simulink model "swGedaempft"  (R2020b)
settings: Solver=ode4  StartTime=0.0  StopTime=30.0  FixedStep=0.1  RelTol=1e-3  EnableMultiTasking=on
settings Model: Creator=Reichl  LastModifiedBy=jakob
settings DataIOCC: LimitDataPoints=on  SaveFormat=Array  SignalLoggingSaveFormat=ModelDataLogs  ReturnWorkspaceOutputs=off
settings OptimizationCC: ExpressionDepthLimit=2147483647  LifeSpan=inf
settings DebuggingCC: UnderspecifiedInitializationDetection=Classic  MergeDetectMultiDrivingBlocksExec=none  SolverPrmCheckMsg=warning  FcnCallInpInsideContextMsg=warning  StateNameClashWarn=warning  SFUnexpectedBacktrackingDiag=warning  SFNoUnconditionalDefaultTransitionDiag=warning  SFExecutionAtInitializationDiag=none  ArithmeticOperatorsInVariantConditions=warning
settings HardwareCC: ProdBitPerPointer=32  ProdBitPerSizeT=32  ProdBitPerPtrDiffT=32  ProdLargestAtomicFloat=None  ProdIntDivRoundTo=Undefined  ProdEndianess=Unspecified  ProdWordSize=32  ProdHWDeviceType=32-bit Generic
settings ModelReferenceCC: PropagateSignalLabelsOutOfModel=off
settings SFSimCC: SimUseLocalCustomCode=off  CustomCodeUndefinedFunction=UseInterfaceOnly
settings RTWCC: RTWUseLocalCustomCode=off
settings CodeAppCC: StateflowObjectComments=on
settings GRTTargetCC: TargetLangStandard=C89/C90 (ANSI)  CombineOutputUpdateFcns=off  GRTInterface=on
settings ConfigComp: CovMetricSettings=dw  CovSaveCumulativeToWorkspaceVar=on  CovSaveSingleToWorkspaceVar=on  CovExternalEMLEnable=off  CovSFcnEnable=off

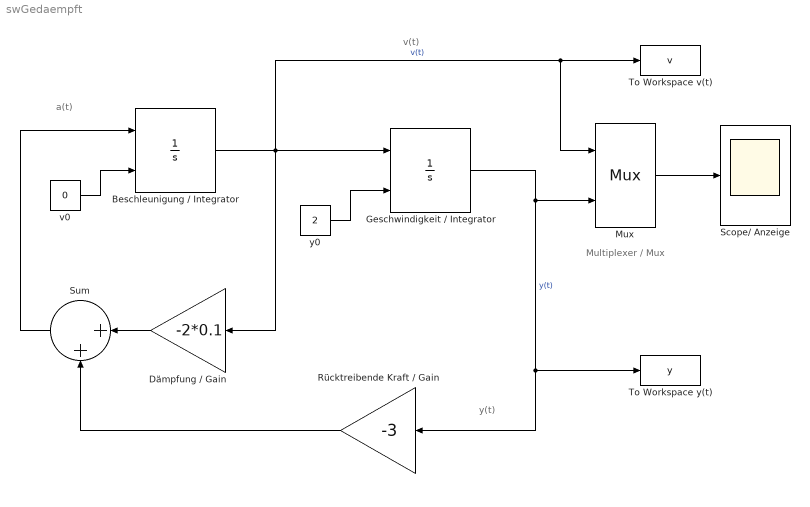
== system swGedaempft ==
  note: v(t)
  note: y(t)
  note: Multiplexer
      |  / Mux
  note: a(t)
  Beschleunigung / Integrator : Integrator  InitialConditionSource=external
  Dämpfung / Gain : Gain  Gain=-2*0.1
  Geschwindigkeit / Integrator : Integrator  InitialConditionSource=external  InitialCondition=3
  Mux : Mux  Inputs=2
      settings: DisplayOption=signals
  Rücktreibende Kraft / Gain : Gain  Gain=-3
  Scope/ Anzeige : Scope
  Sum : Sum  Inputs=|++
  To Workspace v(t) : ToWorkspace  VariableName=v  SampleTime=-1
  To Workspace y(t) : ToWorkspace  VariableName=y  SampleTime=-1
  v0 : Constant  Value=0
  y0 : Constant  Value=2
  wires:
  Beschleunigung / Integrator/1 -> Geschwindigkeit / Integrator/1, Dämpfung / Gain/1, Mux/1, To Workspace v(t)/1  "v(t)"
  Geschwindigkeit / Integrator/1 -> Mux/2, Rücktreibende Kraft / Gain/1, To Workspace y(t)/1  "y(t)"
  Mux/1 -> Scope/ Anzeige/1
  Dämpfung / Gain/1 -> Sum/1
  Rücktreibende Kraft / Gain/1 -> Sum/2
  Sum/1 -> Beschleunigung / Integrator/1
  v0/1 -> Beschleunigung / Integrator/2
  y0/1 -> Geschwindigkeit / Integrator/2
